simulink model "Tires_s"  (R2023a)
settings: Solver=VariableStepAuto  StartTime=0.0  StopTime=10.0  RelTol=1e-3
undefined symbols (not defined in the file): C, C_alpha_f, C_r, E, e_p0, F_zf, l_f, l_r, n_st
settings Model: Creator=Tan_Tram  LastModifiedBy=Tan_Tram

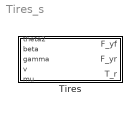
== system Tires_s ==
  Tires : Subsystem

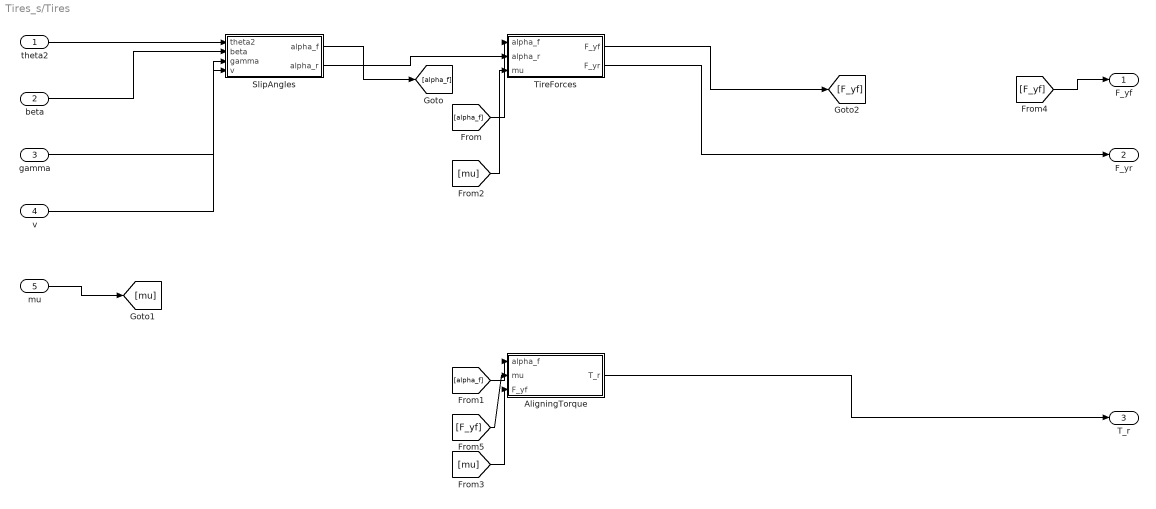
== system Tires_s/Tires ==
  theta2 : Inport
  beta : Inport  Port=2
  gamma : Inport  Port=3
  v : Inport  Port=4
  mu : Inport  Port=5
  AligningTorque : Subsystem
  SlipAngles : Subsystem
  TireForces : Subsystem
  F_yf : Outport
  F_yr : Outport  Port=2
  T_r : Outport  Port=3
  wires:
  theta2/1 -> SlipAngles/1(theta2)
  beta/1 -> SlipAngles/2(beta)
  gamma/1 -> SlipAngles/3(gamma)
  v/1 -> SlipAngles/4(v)
  SlipAngles/1(alpha_f) -> [alpha_f]
  [alpha_f] -> TireForces/1(alpha_f)
  [alpha_f] -> AligningTorque/1(alpha_f)
  SlipAngles/2(alpha_r) -> TireForces/2(alpha_r)
  mu/1 -> [mu]
  [mu] -> TireForces/3(mu)
  [mu] -> AligningTorque/3(F_yf)
  TireForces/1(F_yf) -> [F_yf]
  [F_yf] -> F_yf/1
  [F_yf] -> AligningTorque/2(mu)
  TireForces/2(F_yr) -> F_yr/1
  AligningTorque/1(T_r) -> T_r/1

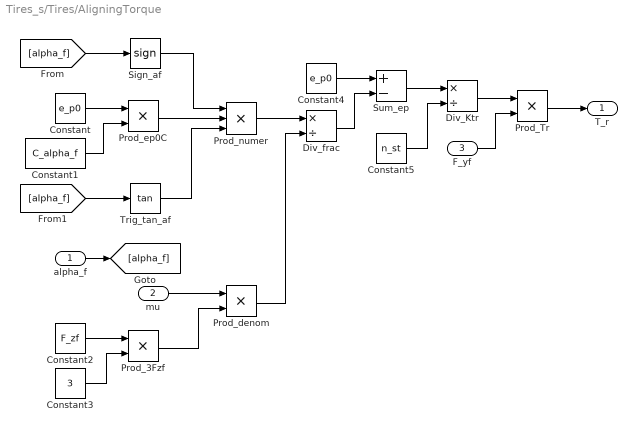
== system Tires_s/Tires/AligningTorque ==
  alpha_f : Inport
  mu : Inport  Port=2
  F_yf : Inport  Port=3
  Constant : Constant  Value=e_p0
  Constant1 : Constant  Value=C_alpha_f
  Constant2 : Constant  Value=F_zf
  Constant3 : Constant  Value=3
  Constant4 : Constant  Value=e_p0
  Constant5 : Constant  Value=n_st
  Div_Ktr : Product  Inputs=*/
  Div_frac : Product  Inputs=*/
  Prod_3Fzf : Product  Inputs=**
  Prod_Tr : Product  Inputs=**
  Prod_denom : Product  Inputs=**
  Prod_ep0C : Product  Inputs=**
  Prod_numer : Product  Inputs=***
  Sign_af : Signum
  Sum_ep : Sum  Inputs=+-
  Trig_tan_af : Trigonometry  Operator=tan
  T_r : Outport
  wires:
  [alpha_f] -> Sign_af/1
  alpha_f/1 -> [alpha_f]
  Constant2/1 -> Prod_3Fzf/1
  Constant/1 -> Prod_ep0C/1
  Sign_af/1 -> Prod_numer/1
  Constant3/1 -> Prod_3Fzf/2
  Constant1/1 -> Prod_ep0C/2
  mu/1 -> Prod_denom/1
  [alpha_f] -> Trig_tan_af/1
  Prod_ep0C/1 -> Prod_numer/2
  Trig_tan_af/1 -> Prod_numer/3
  Prod_3Fzf/1 -> Prod_denom/2
  Prod_denom/1 -> Div_frac/2
  Prod_numer/1 -> Div_frac/1
  Prod_Tr/1 -> T_r/1
  Constant4/1 -> Sum_ep/1
  Div_frac/1 -> Sum_ep/2
  Sum_ep/1 -> Div_Ktr/1
  Constant5/1 -> Div_Ktr/2
  Div_Ktr/1 -> Prod_Tr/1
  F_yf/1 -> Prod_Tr/2

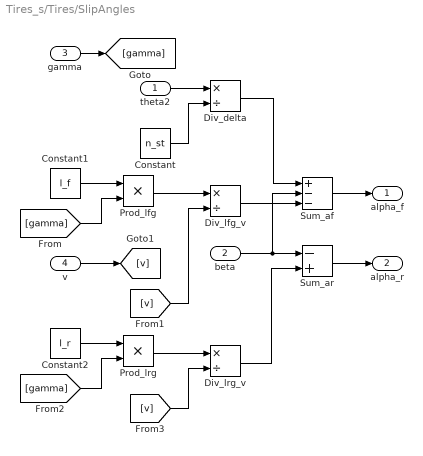
== system Tires_s/Tires/SlipAngles ==
  theta2 : Inport
  beta : Inport  Port=2
  gamma : Inport  Port=3
  v : Inport  Port=4
  Constant : Constant  Value=n_st
  Constant1 : Constant  Value=l_f
  Constant2 : Constant  Value=l_r
  Div_delta : Product  Inputs=*/
  Div_lfg_v : Product  Inputs=*/
  Div_lrg_v : Product  Inputs=*/
  Prod_lfg : Product  Inputs=**
  Prod_lrg : Product  Inputs=**
  Sum_af : Sum  Inputs=+--
  Sum_ar : Sum  Inputs=-+
  alpha_f : Outport
  alpha_r : Outport  Port=2
  wires:
  gamma/1 -> [gamma]
  theta2/1 -> Div_delta/1
  [gamma] -> Prod_lrg/2
  [gamma] -> Prod_lfg/2
  Constant1/1 -> Prod_lfg/1
  v/1 -> [v]
  [v] -> Div_lrg_v/2
  Constant/1 -> Div_delta/2
  Constant2/1 -> Prod_lrg/1
  Div_delta/1 -> Sum_af/1
  Prod_lfg/1 -> Div_lfg_v/1
  [v] -> Div_lfg_v/2
  Div_lfg_v/1 -> Sum_af/3
  Prod_lrg/1 -> Div_lrg_v/1
  beta/1 -> Sum_af/2, Sum_ar/1
  Div_lrg_v/1 -> Sum_ar/2
  Sum_af/1 -> alpha_f/1
  Sum_ar/1 -> alpha_r/1

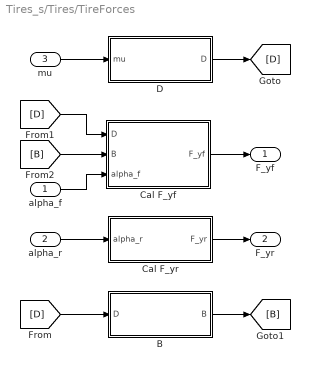
== system Tires_s/Tires/TireForces ==
  alpha_f : Inport
  alpha_r : Inport  Port=2
  mu : Inport  Port=3
  B : Subsystem
  Cal F_yf : Subsystem
  Cal F_yr : Subsystem
  D : Subsystem
  F_yf : Outport
  F_yr : Outport  Port=2
  wires:
  alpha_f/1 -> Cal F_yf/3(alpha_f)
  mu/1 -> D/1(mu)
  D/1(D) -> [D]
  [D] -> Cal F_yf/1(D)
  [D] -> B/1(D)
  [B] -> Cal F_yf/2(B)
  alpha_r/1 -> Cal F_yr/1(alpha_r)
  Cal F_yf/1(F_yf) -> F_yf/1
  B/1(B) -> [B]
  Cal F_yr/1(F_yr) -> F_yr/1

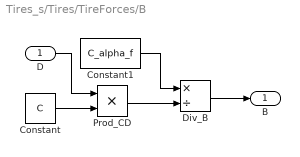
== system Tires_s/Tires/TireForces/B ==
  D : Inport
  Constant : Constant  Value=C
  Constant1 : Constant  Value=C_alpha_f
  Div_B : Product  Inputs=*/
  Prod_CD : Product  Inputs=**
  B : Outport
  wires:
  Constant1/1 -> Div_B/1
  D/1 -> Prod_CD/1
  Div_B/1 -> B/1
  Prod_CD/1 -> Div_B/2
  Constant/1 -> Prod_CD/2

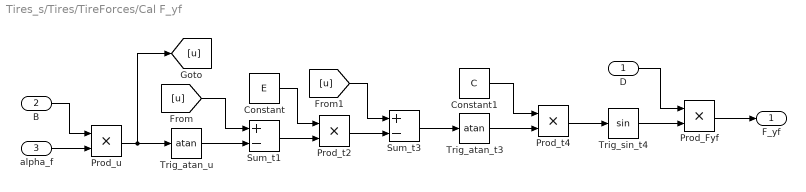
== system Tires_s/Tires/TireForces/Cal F_yf ==
  D : Inport
  B : Inport  Port=2
  alpha_f : Inport  Port=3
  Constant : Constant  Value=E
  Constant1 : Constant  Value=C
  Prod_Fyf : Product  Inputs=**
  Prod_t2 : Product  Inputs=**
  Prod_t4 : Product  Inputs=**
  Prod_u : Product  Inputs=**
  Sum_t1 : Sum  Inputs=+-
  Sum_t3 : Sum  Inputs=+-
  Trig_atan_t3 : Trigonometry  Operator=atan
  Trig_atan_u : Trigonometry  Operator=atan
  Trig_sin_t4 : Trigonometry
  F_yf : Outport
  wires:
  Constant/1 -> Prod_t2/1
  [u] -> Sum_t1/1
  B/1 -> Prod_u/1
  [u] -> Sum_t3/1
  alpha_f/1 -> Prod_u/2
  Trig_atan_u/1 -> Sum_t1/2
  Prod_u/1 -> [u], Trig_atan_u/1
  Sum_t1/1 -> Prod_t2/2
  Prod_t2/1 -> Sum_t3/2
  Sum_t3/1 -> Trig_atan_t3/1
  Constant1/1 -> Prod_t4/1
  Trig_atan_t3/1 -> Prod_t4/2
  Prod_t4/1 -> Trig_sin_t4/1
  D/1 -> Prod_Fyf/1
  Trig_sin_t4/1 -> Prod_Fyf/2
  Prod_Fyf/1 -> F_yf/1

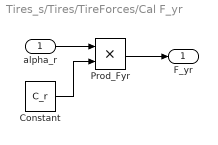
== system Tires_s/Tires/TireForces/Cal F_yr ==
  alpha_r : Inport
  Constant : Constant  Value=C_r
  Prod_Fyr : Product  Inputs=**
  F_yr : Outport
  wires:
  alpha_r/1 -> Prod_Fyr/1
  Prod_Fyr/1 -> F_yr/1
  Constant/1 -> Prod_Fyr/2

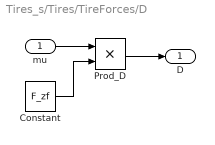
== system Tires_s/Tires/TireForces/D ==
  mu : Inport
  Constant : Constant  Value=F_zf
  Prod_D : Product  Inputs=**
  D : Outport
  wires:
  Prod_D/1 -> D/1
  mu/1 -> Prod_D/1
  Constant/1 -> Prod_D/2
